simulink model "STM32Inverter2Motor"  (R2025a)
settings: Solver=VariableStepAuto  StartTime=0.0  StopTime=10  RelTol=1e-3
model workspace (MAT data in the model file):
  CT_AmpersPerLSB = 0.0515718
  InverterVdc = 440
  Max_ADC_CNT = 4096
  MotorBaseCurrent = 70
  MotorKe = 43.834
  MotorLd = 0.000222
  MotorLq = 0.000355
  MotorPoles = 4
  MotorRs = 0.126
  PID_ramp = 1000
  PI_params_idKi = 1.5
  PI_params_idKp = 1.92
  PI_params_iqKi = 1.5
  PI_params_iqKp = 2.4
  Ts = 4.34782608696e-05
libraries: simulink x2, slpidlib x2, mcbplantlib x1, autolibpmsminterior x1, mcbcontrollergainlib x1, spsRMSLib x1, simulink_extras x1, mcbhdlcontrolslib x1
settings Model: Creator=taiji  LastModifiedBy=taiji
settings DebuggingCC: ParamSuppressDoubleToSinglePrecisionLossMsg=on
settings RTWCC: GenCodeOnly=on  Toolchain=MinGW64 | gmake (64-bit Windows)

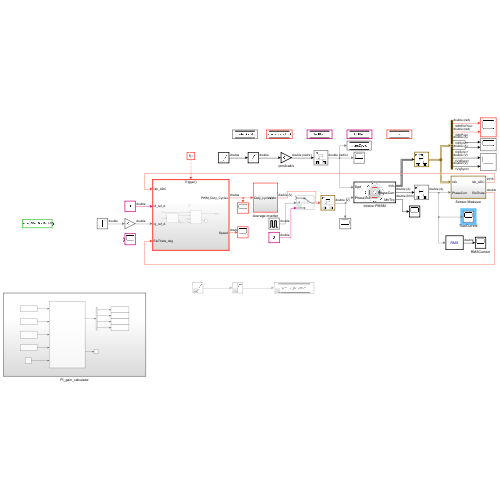
[thumbnail: Simulink's stored preview of the top-level diagram]
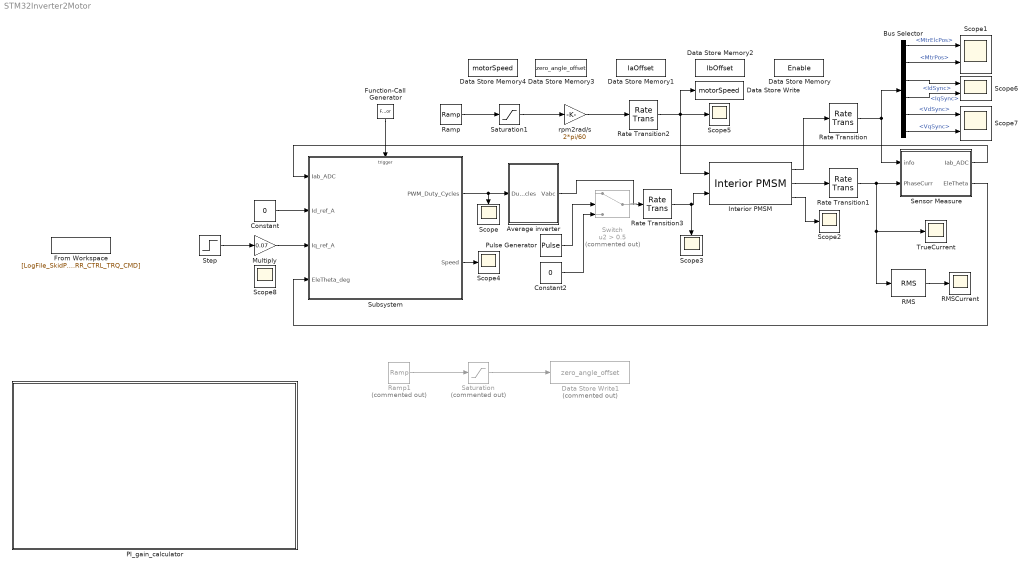
== system STM32Inverter2Motor ==
  Average inverter : Subsystem
  Bus Selector : BusSelector  OutputSignals=MtrElcPos,MtrPos,IdSync,IqSync,VdSync,VqSync
  Constant : Constant  Value=0
  Constant2 : Constant  Value=0
  Data Store Memory : DataStoreMemory  DataStoreName=Enable  WriteAfterWriteMsg=warning  InitialValue=true  ShowAdditionalParam=off  OutDataTypeStr=boolean
  Data Store Memory1 : DataStoreMemory  DataStoreName=IaOffset  WriteAfterWriteMsg=warning  ShowAdditionalParam=off  OutDataTypeStr=boolean
  Data Store Memory2 : DataStoreMemory  DataStoreName=IbOffset  WriteAfterWriteMsg=warning  ShowAdditionalParam=off  OutDataTypeStr=boolean
  Data Store Memory3 : DataStoreMemory  DataStoreName=zero_angle_offset  WriteAfterWriteMsg=warning  InitialValue=36  ShowAdditionalParam=off
  Data Store Memory4 : DataStoreMemory  DataStoreName=motorSpeed  WriteAfterWriteMsg=warning  ShowAdditionalParam=off
  Data Store Write : DataStoreWrite  DataStoreName=motorSpeed  IndexOptions=Index vector (dialog)  Indices=1  OutputSizes=1
  Data Store Write1 : DataStoreWrite  Commented=on  DataStoreName=zero_angle_offset  IndexOptions=Index vector (dialog)  Indices=1  OutputSizes=1
  From Workspace : FromWorkspace  VariableName=[LogFile_SkidPadHiL_TCon_TCoff_0825.Time LogFile_SkidPadHiL_TCon_TCoff_0825.RR_CTRL_TRQ_CMD]  SampleTime=0.001
  Function-Call Generator : FunctionCallGenerator  SampleTime=Ts
  Interior PMSM : autolibpmsminterior/Interior PMSM  port_config=Speed  sim_type=Continuous  Ts=Ts  P=MotorPoles  Rs=MotorRs  Ldq=[MotorLd MotorLq]  KConstText=Back-emf constant (Ke):  lambda_pm=0.0427  Ke=MotorKe  mechanical=[0.33e-3,4.924e-4,0]  idq0=[0 0]  theta_init=0  omega_init=0  KConst=MotorKe  lambda_pm_calc=0.060417  Kt=0.07  RefBlkName='autolibpmsminterior/Interior PMSM'  aMode=5
      settings: LibrarySourceBlock=mcblib/Electrical Systems/Motors/Interior PMSM
  Multiply : Gain  Gain=0.07
  PI_gain_calculator : Subsystem
  Pulse Generator : DiscretePulseGenerator  PulseType=Time based  Period=0.01  PulseWidth=99.99
  RMS : spsRMSLib/RMS  TrueRMS=on  Freq=10  RMSInit=1  Ts=0
  RMSCurrent : Scope
      settings: ActiveDisplayYMinimum=-1  ActiveDisplayYMaximum=1
  Ramp : simulink/Sources/Ramp  slope=100  start=1  InitialOutput=0
  Ramp1 : simulink/Sources/Ramp  Commented=on  slope=36  start=1  InitialOutput=0
  Rate Transition{,1..3} (4 alike) : RateTransition
  Saturation : Saturate  Commented=on  UpperLimit=360  LowerLimit=0
  Saturation1 : Saturate  UpperLimit=600  LowerLimit=0
  Scope{,2..5,8} (6 alike) : Scope
      Scope settings: ActiveDisplayYMinimum=0.15237461254211696  ActiveDisplayYMaximum=0.847625387457883
      Scope2 settings: ActiveDisplayYMinimum=-45.081836654015575  ActiveDisplayYMaximum=14.201489134555768  DataLoggingVariableName=ScopeData2
      Scope3 settings: ActiveDisplayYMinimum=-253.21724341215781  ActiveDisplayYMaximum=253.44594110211258  DataLoggingVariableName=ScopeData3
      Scope4 settings: ActiveDisplayYMinimum=-1  ActiveDisplayYMaximum=1  DataLoggingVariableName=ScopeData2
      Scope5 settings: ActiveDisplayYMinimum=-1  ActiveDisplayYMaximum=1  DataLoggingVariableName=ScopeData9
      Scope8 settings: ActiveDisplayYMinimum=-1  ActiveDisplayYMaximum=1  DataLoggingVariableName=ScopeData14
  Scope1 : Scope  NumInputPorts=2
      settings: ActiveDisplayYMinimum=-1  ActiveDisplayYMaximum=1
  Scope6 : Scope  NumInputPorts=2
  Scope7 : Scope  NumInputPorts=2
      settings: ActiveDisplayYMinimum=-0.8281  ActiveDisplayYMaximum=6.44112  DataLoggingVariableName=ScopeData2
  Sensor Measure : Subsystem
  Step : Step  Time=0.2  After=1000  SampleTime=0
  Subsystem : Subsystem
  Switch : Switch  Commented=on  Criteria=u2 > Threshold  Threshold=0.5  SaturateOnIntegerOverflow=off  InputSameDT=off
  TrueCurrent : Scope
      settings: ActiveDisplayYMinimum=-87.035051528006122  ActiveDisplayYMaximum=87.028426331999526  DataLoggingVariableName=ScopeData7
  rpm2rad/s : Gain  Gain=2*pi/60
  wires:
  Interior PMSM/1 -> Rate Transition/1
  Interior PMSM/2 -> Rate Transition1/1
  Average inverter/1(Vabc) -> Rate Transition3/1
  Rate Transition/1 -> Sensor Measure/1(info), Bus Selector/1
  Rate Transition1/1 -> RMS/1, TrueCurrent/1, Sensor Measure/2(PhaseCurr)
  Bus Selector/1 -> Scope1/1  "<MtrElcPos>"
  Rate Transition3/1 -> Interior PMSM/2, Scope3/1
  Function-Call Generator/1 -> Subsystem/Trigger
  Subsystem/1(PWM_Duty_Cycles) -> Average inverter/1(Duty_cycles), Scope/1
  Interior PMSM/3 -> Scope2/1
  RMS/1 -> RMSCurrent/1
  Subsystem/2(Speed) -> Scope4/1
  Ramp/1 -> Saturation1/1
  Rate Transition2/1 -> Interior PMSM/1, Data Store Write/1, Scope5/1
  rpm2rad/s/1 -> Rate Transition2/1
  Bus Selector/2 -> Scope1/2  "<MtrPos>"
  Bus Selector/3 -> Scope6/1  "<IdSync>"
  Bus Selector/4 -> Scope6/2  "<IqSync>"
  Bus Selector/5 -> Scope7/1  "<VdSync>"
  Bus Selector/6 -> Scope7/2  "<VqSync>"
  Constant/1 -> Subsystem/2(Id_ref_A)
  Multiply/1 -> Subsystem/3(Iq_ref_A)
  Ramp1/1 -> Saturation/1
  Sensor Measure/2(EleTheta) -> Subsystem/4(EleTheta_deg)
  Sensor Measure/1(Iab_ADC) -> Subsystem/1(Iab_ADC)
  Saturation/1 -> Data Store Write1/1
  Saturation1/1 -> rpm2rad/s/1
  Switch/1 -> ?
  Pulse Generator/1 -> Switch/2
  Constant2/1 -> Switch/3
  Step/1 -> Multiply/1

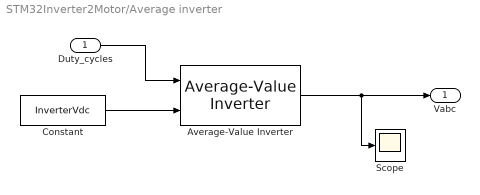
== system STM32Inverter2Motor/Average inverter ==
  Duty_cycles : Inport
  Average-Value Inverter : mcbplantlib/Average-Value Inverter
      settings: LibrarySourceBlock=mcblib/Electrical Systems/Inverters/Average-Value Inverter
  Constant : Constant  Value=InverterVdc
  Scope : Scope
      settings: ActiveDisplayYMinimum=-313.23796592607141  ActiveDisplayYMaximum=350.5718291969751  DataLoggingVariableName=ScopeData6
  Vabc : Outport
  wires:
  Duty_cycles/1 -> Average-Value Inverter/1
  Constant/1 -> Average-Value Inverter/2
  Average-Value Inverter/1 -> Scope/1, Vabc/1

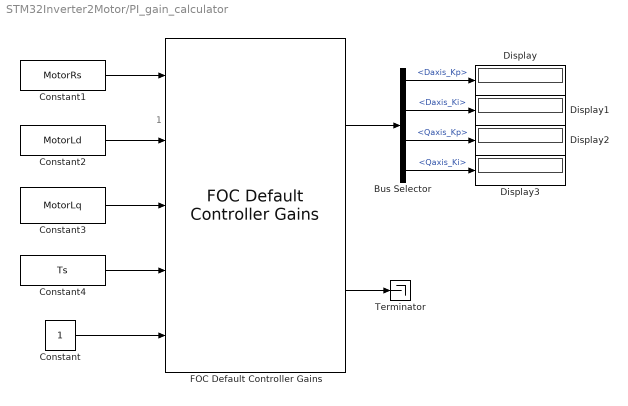
== system STM32Inverter2Motor/PI_gain_calculator ==
  note: 1
  Bus Selector : BusSelector  OutputSignals=Daxis_Kp,Daxis_Ki,Qaxis_Kp,Qaxis_Ki
  Constant : Constant
  Constant1 : Constant  Value=MotorRs
  Constant2 : Constant  Value=MotorLd
  Constant3 : Constant  Value=MotorLq
  Constant4 : Constant  Value=Ts  VectorParams1D=off
  Display{,1..3} (4 alike) : Display
  FOC Default Controller Gains : mcbcontrollergainlib/FOC Default Controller Gains  ControllerGainType=Empirical method  motorSelection=PMSM  unitType=SI Unit  outCurrentControlGain=on  outFWCGain=off  outSpeedControlGain=off  externalDelay=off  currentSensorDelay=50e-6  speedSensorDelay=50e-6  speedFilterDelay=0.02
      settings: LibrarySourceBlock=mcblib/Controls/Controllers/FOC Default Controller Gains
  Terminator : Terminator
  wires:
  FOC Default Controller Gains/1 -> Bus Selector/1
  FOC Default Controller Gains/2 -> Terminator/1
  Constant4/1 -> FOC Default Controller Gains/4
  Constant3/1 -> FOC Default Controller Gains/3
  Constant2/1 -> FOC Default Controller Gains/2
  Constant1/1 -> FOC Default Controller Gains/1
  Constant/1 -> FOC Default Controller Gains/5
  Bus Selector/1 -> Display/1  "<Daxis_Kp>"
  Bus Selector/2 -> Display1/1  "<Daxis_Ki>"
  Bus Selector/3 -> Display2/1  "<Qaxis_Kp>"
  Bus Selector/4 -> Display3/1  "<Qaxis_Ki>"

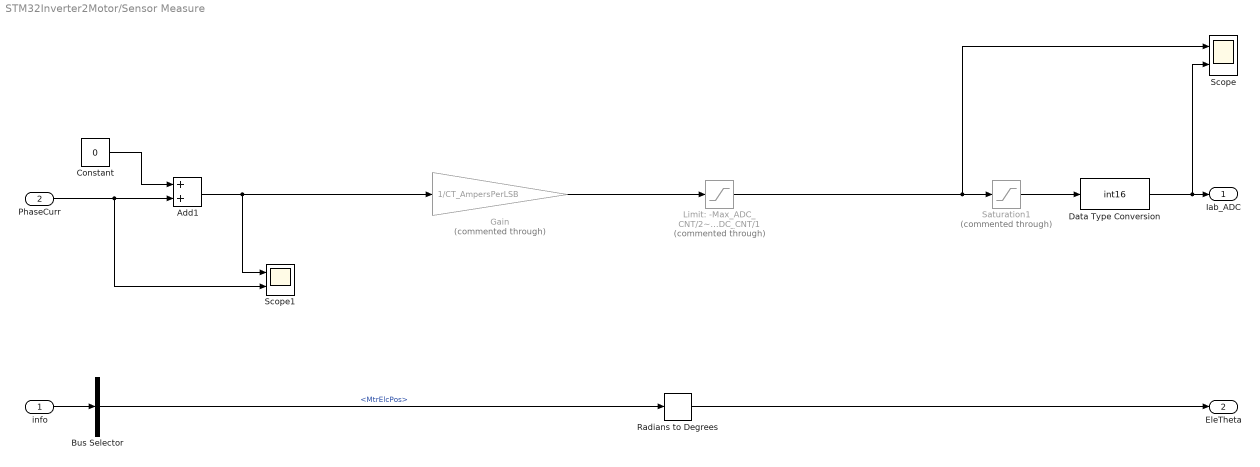
== system STM32Inverter2Motor/Sensor Measure ==
  info : Inport
  PhaseCurr : Inport  Port=2
  Add1 : Sum
  Bus Selector : BusSelector  OutputSignals=MtrElcPos
  Constant : Constant  Value=0
  Data Type Conversion : DataTypeConversion  OutDataTypeStr=int16  SaturateOnIntegerOverflow=off  RndMeth=Floor
  Gain : Gain  Commented=through  Gain=1/CT_AmpersPerLSB
  Limit: -Max_ADC_CNT/2~Max_ADC_CNT/1 : Saturate  Commented=through  UpperLimit=Max_ADC_CNT/2  LowerLimit=-Max_ADC_CNT/2
  Radians to Degrees : simulink_extras/Transformations/Radians to Degrees
  Saturation1 : Saturate  Commented=through  UpperLimit=Max_ADC_CNT  LowerLimit=0
  Scope : Scope  NumInputPorts=2
      settings: ActiveDisplayYMinimum=-2386.1587583821911  ActiveDisplayYMaximum=2388.3518252217932
  Scope1 : Scope  NumInputPorts=2
      settings: ActiveDisplayYMinimum=-2421.1249474633973  ActiveDisplayYMaximum=2418.5627534419714
  Iab_ADC : Outport
  EleTheta : Outport  Port=2
  wires:
  Gain/1 -> Limit: -Max_ADC_CNT/2~Max_ADC_CNT/1/1
  Saturation1/1 -> Data Type Conversion/1
  Limit: -Max_ADC_CNT/2~Max_ADC_CNT/1/1 -> Scope/1, Saturation1/1
  Add1/1 -> Scope1/1, Gain/1
  Data Type Conversion/1 -> Scope/2, Iab_ADC/1
  info/1 -> Bus Selector/1
  Bus Selector/1 -> Radians to Degrees/1  "<MtrElcPos>"
  PhaseCurr/1 -> Scope1/2, Add1/2
  Constant/1 -> Add1/1
  Radians to Degrees/1 -> EleTheta/1

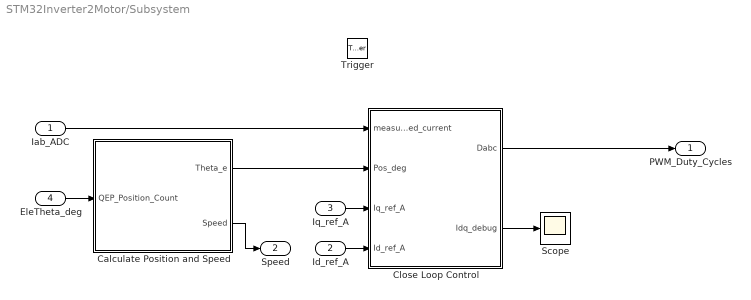
== system STM32Inverter2Motor/Subsystem ==
  Iab_ADC : Inport
  Id_ref_A : Inport  Port=2
  Iq_ref_A : Inport  Port=3
  EleTheta_deg : Inport  Port=4
  Trigger : TriggerPort  TriggerType=function-call  VariantControl=(inherit)  PortDimensions=1
  Calculate Position and Speed : Subsystem
  Close Loop Control : Subsystem
  Scope : Scope
      settings: ActiveDisplayYMinimum=-1  ActiveDisplayYMaximum=1  DataLoggingVariableName=ScopeData8
  PWM_Duty_Cycles : Outport
  Speed : Outport  Port=2
  wires:
  Calculate Position and Speed/1(Theta_e) -> Close Loop Control/2(Pos_deg)
  Iab_ADC/1 -> Close Loop Control/1(measured_current)
  Close Loop Control/1(Dabc) -> PWM_Duty_Cycles/1
  Close Loop Control/2(Idq_debug) -> Scope/1
  Calculate Position and Speed/2(Speed) -> Speed/1
  EleTheta_deg/1 -> Calculate Position and Speed/1(QEP_Position_Count)
  Iq_ref_A/1 -> Close Loop Control/3(Iq_ref_A)
  Id_ref_A/1 -> Close Loop Control/4(Id_ref_A)

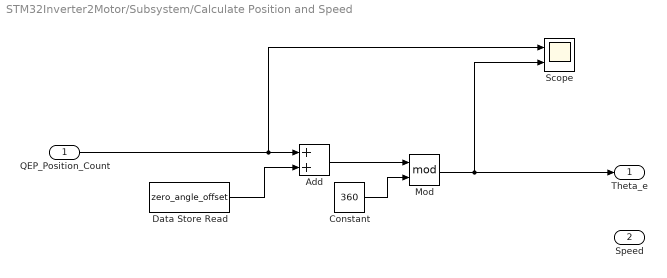
== system STM32Inverter2Motor/Subsystem/Calculate Position and Speed ==
  QEP_Position_Count : Inport
  Add : Sum
  Constant : Constant  Value=360
  Data Store Read : DataStoreRead  DataStoreName=zero_angle_offset  IndexOptions=Index vector (dialog)  Indices=1  OutputSizes=1
  Mod : Math  Operator=mod
  Scope : Scope  NumInputPorts=2
      settings: ActiveDisplayYMinimum=-1  ActiveDisplayYMaximum=1
  Theta_e : Outport
  Speed : Outport  Port=2
  wires:
  QEP_Position_Count/1 -> Scope/1, Add/1
  Constant/1 -> Mod/2
  Add/1 -> Mod/1
  Data Store Read/1 -> Add/2
  Mod/1 -> Theta_e/1, Scope/2

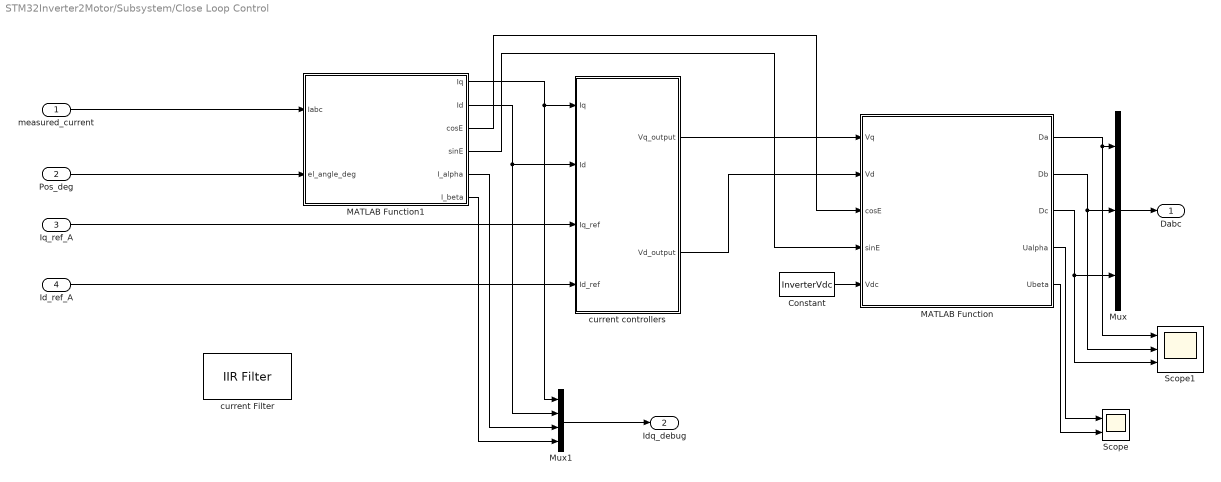
== system STM32Inverter2Motor/Subsystem/Close Loop Control ==
  measured_current : Inport
  Pos_deg : Inport  Port=2
  Iq_ref_A : Inport  Port=3
  Id_ref_A : Inport  Port=4
  Constant : Constant  Value=InverterVdc
  MATLAB Function : MATLAB Function  TreatAsAtomicUnit=on
  MATLAB Function1 : MATLAB Function  TreatAsAtomicUnit=on
  Mux : Mux  Inputs=3
  Mux1 : Mux
  Scope : Scope  NumInputPorts=2
      settings: ActiveDisplayYMinimum=-1  ActiveDisplayYMaximum=1  DataLoggingVariableName=ScopeData11
  Scope1 : Scope  NumInputPorts=3
      settings: ActiveDisplayYMinimum=-0.12499999999999997  ActiveDisplayYMaximum=1.125
  current Filter : mcbhdlcontrolslib/IIR Filter  VariantControl=Low Pass Filter  VariantSelect=Low-pass  FilterConstantInputType=Specify via dialog  Filter_constant=0.532  advancedSettings=on  Ts=Ts  cutOff_freq=4161.1536
      settings: LibrarySourceBlock=mcbhdllib/Signal Management/IIR Filter
  current controllers : Subsystem
  Dabc : Outport
  Idq_debug : Outport  Port=2
  wires:
  MATLAB Function1/2(Id) -> Mux1/2, current controllers/2(Id)
  Iq_ref_A/1 -> current controllers/3(Iq_ref)
  Mux/1 -> Dabc/1
  MATLAB Function1/1(Iq) -> Mux1/1, current controllers/1(Iq)
  Id_ref_A/1 -> current controllers/4(Id_ref)
  Mux1/1 -> Idq_debug/1
  MATLAB Function/1(Da) -> Mux/1, Scope1/1
  MATLAB Function/2(Db) -> Mux/2, Scope1/2
  MATLAB Function/3(Dc) -> Mux/3, Scope1/3
  measured_current/1 -> MATLAB Function1/1(Iabc)
  Pos_deg/1 -> MATLAB Function1/2(el_angle_deg)
  Constant/1 -> MATLAB Function/5(Vdc)
  current controllers/1(Vq_output) -> MATLAB Function/1(Vq)
  current controllers/2(Vd_output) -> MATLAB Function/2(Vd)
  MATLAB Function1/3(cosE) -> MATLAB Function/3(cosE)
  MATLAB Function1/4(sinE) -> MATLAB Function/4(sinE)
  MATLAB Function1/5(I_alpha) -> Mux1/3
  MATLAB Function1/6(I_beta) -> Mux1/4
  MATLAB Function/4(Ualpha) -> Scope/1
  MATLAB Function/5(Ubeta) -> Scope/2

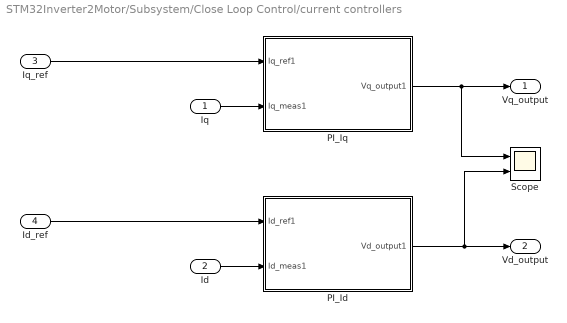
== system STM32Inverter2Motor/Subsystem/Close Loop Control/current controllers ==
  Iq : Inport
  Id : Inport  Port=2
  Iq_ref : Inport  Port=3
  Id_ref : Inport  Port=4
  PI_Id : Subsystem
  PI_Iq : Subsystem
  Scope : Scope  NumInputPorts=2
      settings: ActiveDisplayYMinimum=-1  ActiveDisplayYMaximum=1  DataLoggingVariableName=ScopeData12
  Vq_output : Outport
  Vd_output : Outport  Port=2
  wires:
  PI_Iq/1(Vq_output1) -> Vq_output/1, Scope/1
  PI_Id/1(Vd_output1) -> Scope/2, Vd_output/1
  Id/1 -> PI_Id/2(Id_meas1)
  Iq/1 -> PI_Iq/2(Iq_meas1)
  Iq_ref/1 -> PI_Iq/1(Iq_ref1)
  Id_ref/1 -> PI_Id/1(Id_ref1)

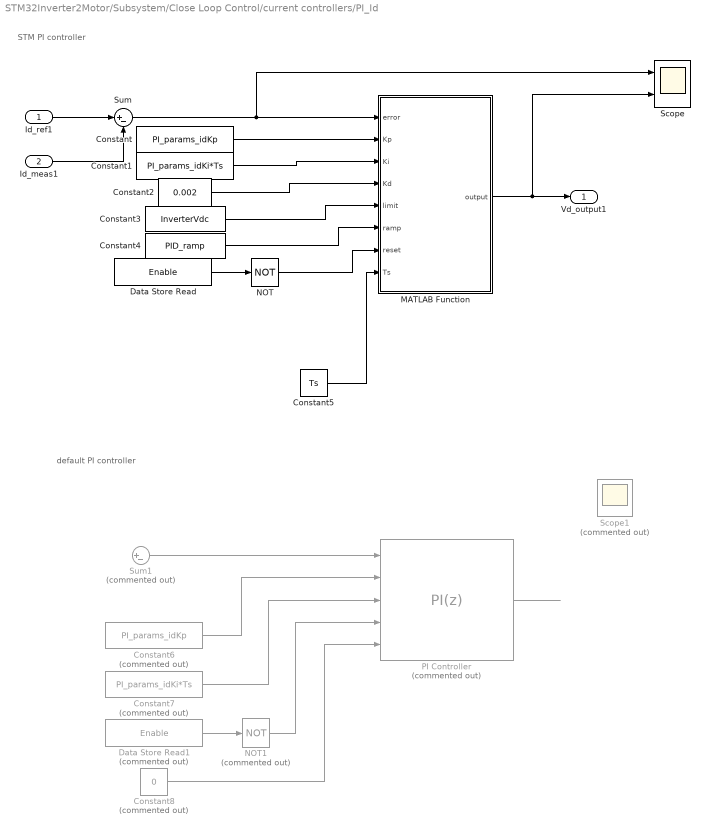
== system STM32Inverter2Motor/Subsystem/Close Loop Control/current controllers/PI_Id ==
  note: STM PI controller
  note: default PI controller
  Id_ref1 : Inport
  Id_meas1 : Inport  Port=2
  Constant : Constant  Value=PI_params_idKp
  Constant1 : Constant  Value=PI_params_idKi*Ts
  Constant2 : Constant  Value=0.002
  Constant3 : Constant  Value=InverterVdc
  Constant4 : Constant  Value=PID_ramp
  Constant5 : Constant  Value=Ts
  Constant6 : Constant  Commented=on  Value=PI_params_idKp
  Constant7 : Constant  Commented=on  Value=PI_params_idKi*Ts
  Constant8 : Constant  Commented=on  Value=0
  Data Store Read : DataStoreRead  DataStoreName=Enable  IndexOptions=Index vector (dialog)  Indices=1  OutputSizes=1
  Data Store Read1 : DataStoreRead  Commented=on  DataStoreName=Enable  IndexOptions=Index vector (dialog)  Indices=1  OutputSizes=1
  MATLAB Function : MATLAB Function  TreatAsAtomicUnit=on
  NOT : Logic  Operator=NOT  IconShape=distinctive  AllPortsSameDT=off  OutDataTypeStr=boolean
  NOT1 : Logic  Commented=on  Operator=NOT  IconShape=distinctive  AllPortsSameDT=off  OutDataTypeStr=boolean
  PI Controller : slpidlib/PID Controller  Commented=on  Controller=PI  Form=Parallel  TimeDomain=Discrete-time  UseExternalTs=off  SampleTime=-1  IntegratorMethod=Forward Euler  FilterMethod=Forward Euler  ControllerParametersSource=external  P=1  I=1  UseKiTs=on  D=0  UseExternalDerivativeSource=off  N=100  UseFilter=on  TunerSelectOption=Transfer Function Based (PID Tuner App)  InitialConditionSource=external  InitialConditionForIntegrator=0  InitialConditionForFilter=0  DifferentiatorICPrevScaledInput=0  ExternalReset=level  TrackingMode=off  Kt=1  LimitOutput=on  SatLimitsSource=internal  UpperSaturationLimit=InverterVdc  LowerSaturationLimit=-InverterVdc  LinearizeAsGain=on  AntiWindupMode=clamping  Kb=1  LimitIntegrator=on  UpperIntegratorSaturationLimit=InverterVdc  LowerIntegratorSaturationLimit=-InverterVdc  RndMeth=Simplest  POutMin=[]  POutMax=[]  IOutMin=[]  IOutMax=[]  DOutMin=[]  DOutMax=[]  NOutMin=[]  NOutMax=[]  SumOutMin=[]  SumOutMax=[]  SaturationOutDataTypeStr=Inherit: Inherit via back propagation  SaturationOutMin=[]  SaturationOutMax=[]  PParamMin=[]  PParamMax=[]  IParamMin=[]  IParamMax=[]  DParamMin=[]  DParamMax=[]  NParamMin=[]  NParamMax=[]  KbParamMin=[]  KbParamMax=[]  KtParamMin=[]  KtParamMax=[]  KbOutMin=[]  KbOutMax=[]  KtOutMin=[]  KtOutMax=[]  IntegratorOutMin=[]  IntegratorOutMax=[]  FilterOutMin=[]  FilterOutMax=[]  SumI1OutMin=[]  SumI1OutMax=[]  SumI2OutMin=[]  SumI2OutMax=[]  SumI3OutMin=[]  SumI3OutMax=[]  SumI4OutMin=[]  SumI4OutMax=[]  SumDOutMin=[]  SumDOutMax=[]  DifferentiatorOutMin=[]  DifferentiatorOutMax=[]  FilterDiffOutCoefMin=[]  FilterDiffOutCoefMax=[]  ReciprocalOutMin=[]  ReciprocalOutMax=[]  SumDenOutMin=[]  SumDenOutMax=[]  SumNumOutMin=[]  SumNumOutMax=[]  DivideOutMin=[]  DivideOutMax=[]  UdiffTsProdOutMin=[]  UdiffTsProdOutMax=[]  NTsProdOutMin=[]  NTsProdOutMax=[]  UintegralTsProdOutMin=[]  UintegralTsProdOutMax=[]  UngainTsProdOutMin=[]  UngainTsProdOutMax=[]  ClampingZeroOutDataTypeStr=Inherit: Inherit via back propagation  ClampingZeroOutMin=[]  ClampingZeroOutMax=[]  FilterDenConstantOutDataTypeStr=Inherit: Inherit via back propagation  FilterDenConstantOutMin=[]  FilterDenConstantOutMax=[]  PCopyOutDataTypeStr=Inherit: Inherit via back propagation  PCopyOutMin=[]  PCopyOutMax=[]  NCopyOutDataTypeStr=Inherit: Inherit via back propagation  NCopyOutMin=[]  NCopyOutMax=[]  IntegratorContinuousStateAttributes=''  IntegratorStateMustResolveToSignalObject=off  IntegratorRTWStateStorageClass=Auto  FilterContinuousStateAttributes=''  FilterStateMustResolveToSignalObject=off  FilterRTWStateStorageClass=Auto  ParallelPVariant=ExternalParameters  IdealPVariant=Disabled  IVariant=ExternalParameters  DVariant=Disabled  IntegratorVariant=Discrete  SatVariant=Enabled  AWVariant=DiscClampingParallel  PCopyVariant=Disabled  TRVariant=Disabled  FdbkBlocksVariant=Forward  IdealPFdbkVariant=Disabled  SatFdbkVariant=Disabled  DerivativeFilterVariant=Disabled  NVariant=Disabled  NCopyVariant=Disabled_SignalSpec  FilterICVariant=Disabled  IntegratorICVariant=ExternalICs  ExternalResetVariant=ExternalReset  TRSumVariant=Passthrough  SumFdbkVariant=Disabled  SumVariant=Sum_PI  TsampFilterVariant=InternalTs  TsampNgainVariant=Passthrough  TsampIntegralVariant=Disabled_SignalSpec  ExternalSaturationOutDataTypeStr=Inherit: Same as second input  DerivativeSourceVariant=Disabled  PreIntVariant=InternalPreInt
  Scope : Scope  NumInputPorts=2
      settings: ActiveDisplayYMinimum=-4.2718355978255875  ActiveDisplayYMaximum=8.44652038043029  DataLoggingVariableName=ScopeData10
  Scope1 : Scope  Commented=on  NumInputPorts=3
      settings: ActiveDisplayYMinimum=-1  ActiveDisplayYMaximum=1  DataLoggingVariableName=ScopeData15
  Sum : Sum  Inputs=|+-
  Sum1 : Sum  Commented=on  Inputs=|+-
  Vd_output1 : Outport
  wires:
  Id_ref1/1 -> Sum/1
  Constant2/1 -> MATLAB Function/4(Kd)
  NOT/1 -> MATLAB Function/7(reset)
  Id_meas1/1 -> Sum/2
  Constant1/1 -> MATLAB Function/3(Ki)
  Constant/1 -> MATLAB Function/2(Kp)
  Data Store Read/1 -> NOT/1
  Sum/1 -> Scope/1, MATLAB Function/1(error)
  Constant3/1 -> MATLAB Function/5(limit)
  Constant4/1 -> MATLAB Function/6(ramp)
  Constant5/1 -> MATLAB Function/8(Ts)
  MATLAB Function/1(output) -> Vd_output1/1, Scope/2
  ? -> Scope1/2, Sum1/2
  Data Store Read1/1 -> NOT1/1
  Constant7/1 -> PI Controller/3
  ? -> Scope1/1, Sum1/1
  Constant6/1 -> PI Controller/2
  Constant8/1 -> PI Controller/5
  NOT1/1 -> PI Controller/4
  Sum1/1 -> PI Controller/1
  PI Controller/1 -> ?

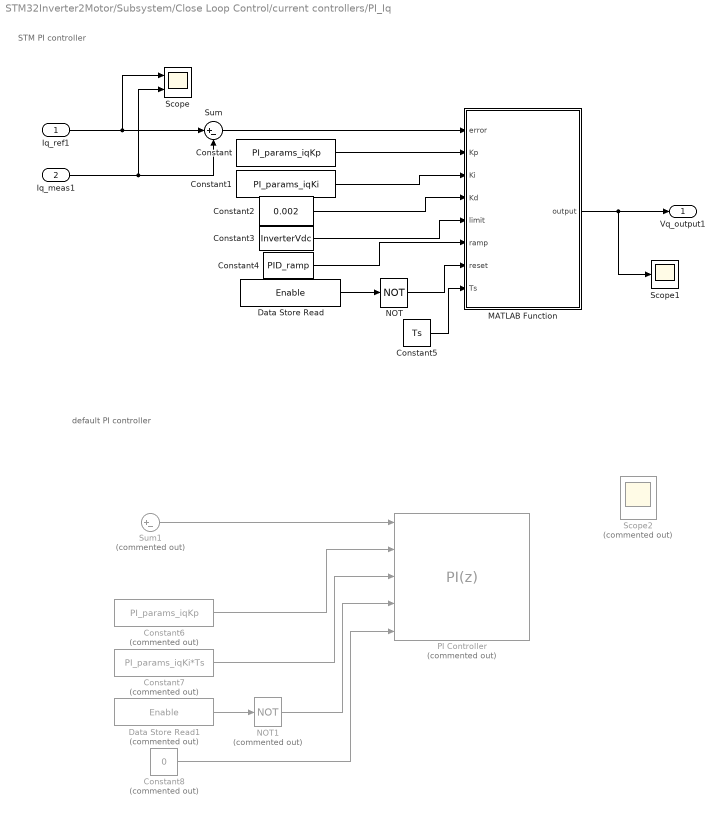
== system STM32Inverter2Motor/Subsystem/Close Loop Control/current controllers/PI_Iq ==
  note: STM PI controller
  note: default PI controller
  Iq_ref1 : Inport
  Iq_meas1 : Inport  Port=2
  Constant : Constant  Value=PI_params_iqKp
  Constant1 : Constant  Value=PI_params_iqKi
  Constant2 : Constant  Value=0.002
  Constant3 : Constant  Value=InverterVdc
  Constant4 : Constant  Value=PID_ramp
  Constant5 : Constant  Value=Ts
  Constant6 : Constant  Commented=on  Value=PI_params_iqKp
  Constant7 : Constant  Commented=on  Value=PI_params_iqKi*Ts
  Constant8 : Constant  Commented=on  Value=0
  Data Store Read : DataStoreRead  DataStoreName=Enable  IndexOptions=Index vector (dialog)  Indices=1  OutputSizes=1
  Data Store Read1 : DataStoreRead  Commented=on  DataStoreName=Enable  IndexOptions=Index vector (dialog)  Indices=1  OutputSizes=1
  MATLAB Function : MATLAB Function  TreatAsAtomicUnit=on
  NOT : Logic  Operator=NOT  IconShape=distinctive  AllPortsSameDT=off  OutDataTypeStr=boolean
  NOT1 : Logic  Commented=on  Operator=NOT  IconShape=distinctive  AllPortsSameDT=off  OutDataTypeStr=boolean
  PI Controller : slpidlib/PID Controller  Commented=on  Controller=PI  Form=Parallel  TimeDomain=Discrete-time  UseExternalTs=off  SampleTime=-1  IntegratorMethod=Forward Euler  FilterMethod=Forward Euler  ControllerParametersSource=external  P=1  I=1  UseKiTs=on  D=0  UseExternalDerivativeSource=off  N=100  UseFilter=on  TunerSelectOption=Transfer Function Based (PID Tuner App)  InitialConditionSource=external  InitialConditionForIntegrator=0  InitialConditionForFilter=0  DifferentiatorICPrevScaledInput=0  ExternalReset=level  TrackingMode=off  Kt=1  LimitOutput=on  SatLimitsSource=internal  UpperSaturationLimit=InverterVdc  LowerSaturationLimit=-InverterVdc  LinearizeAsGain=on  AntiWindupMode=clamping  Kb=1  LimitIntegrator=on  UpperIntegratorSaturationLimit=InverterVdc  LowerIntegratorSaturationLimit=-InverterVdc  RndMeth=Simplest  POutMin=[]  POutMax=[]  IOutMin=[]  IOutMax=[]  DOutMin=[]  DOutMax=[]  NOutMin=[]  NOutMax=[]  SumOutMin=[]  SumOutMax=[]  SaturationOutDataTypeStr=Inherit: Inherit via back propagation  SaturationOutMin=[]  SaturationOutMax=[]  PParamMin=[]  PParamMax=[]  IParamMin=[]  IParamMax=[]  DParamMin=[]  DParamMax=[]  NParamMin=[]  NParamMax=[]  KbParamMin=[]  KbParamMax=[]  KtParamMin=[]  KtParamMax=[]  KbOutMin=[]  KbOutMax=[]  KtOutMin=[]  KtOutMax=[]  IntegratorOutMin=[]  IntegratorOutMax=[]  FilterOutMin=[]  FilterOutMax=[]  SumI1OutMin=[]  SumI1OutMax=[]  SumI2OutMin=[]  SumI2OutMax=[]  SumI3OutMin=[]  SumI3OutMax=[]  SumI4OutMin=[]  SumI4OutMax=[]  SumDOutMin=[]  SumDOutMax=[]  DifferentiatorOutMin=[]  DifferentiatorOutMax=[]  FilterDiffOutCoefMin=[]  FilterDiffOutCoefMax=[]  ReciprocalOutMin=[]  ReciprocalOutMax=[]  SumDenOutMin=[]  SumDenOutMax=[]  SumNumOutMin=[]  SumNumOutMax=[]  DivideOutMin=[]  DivideOutMax=[]  UdiffTsProdOutMin=[]  UdiffTsProdOutMax=[]  NTsProdOutMin=[]  NTsProdOutMax=[]  UintegralTsProdOutMin=[]  UintegralTsProdOutMax=[]  UngainTsProdOutMin=[]  UngainTsProdOutMax=[]  ClampingZeroOutDataTypeStr=Inherit: Inherit via back propagation  ClampingZeroOutMin=[]  ClampingZeroOutMax=[]  FilterDenConstantOutDataTypeStr=Inherit: Inherit via back propagation  FilterDenConstantOutMin=[]  FilterDenConstantOutMax=[]  PCopyOutDataTypeStr=Inherit: Inherit via back propagation  PCopyOutMin=[]  PCopyOutMax=[]  NCopyOutDataTypeStr=Inherit: Inherit via back propagation  NCopyOutMin=[]  NCopyOutMax=[]  IntegratorContinuousStateAttributes=''  IntegratorStateMustResolveToSignalObject=off  IntegratorRTWStateStorageClass=Auto  FilterContinuousStateAttributes=''  FilterStateMustResolveToSignalObject=off  FilterRTWStateStorageClass=Auto  ParallelPVariant=ExternalParameters  IdealPVariant=Disabled  IVariant=ExternalParameters  DVariant=Disabled  IntegratorVariant=Discrete  SatVariant=Enabled  AWVariant=DiscClampingParallel  PCopyVariant=Disabled  TRVariant=Disabled  FdbkBlocksVariant=Forward  IdealPFdbkVariant=Disabled  SatFdbkVariant=Disabled  DerivativeFilterVariant=Disabled  NVariant=Disabled  NCopyVariant=Disabled_SignalSpec  FilterICVariant=Disabled  IntegratorICVariant=ExternalICs  ExternalResetVariant=ExternalReset  TRSumVariant=Passthrough  SumFdbkVariant=Disabled  SumVariant=Sum_PI  TsampFilterVariant=InternalTs  TsampNgainVariant=Passthrough  TsampIntegralVariant=Disabled_SignalSpec  ExternalSaturationOutDataTypeStr=Inherit: Same as second input  DerivativeSourceVariant=Disabled  PreIntVariant=InternalPreInt
      settings: LibrarySourceBlock=mcblib/Controls/Controllers/PI Controller
  Scope : Scope  NumInputPorts=2
      settings: ActiveDisplayYMinimum=-8.9999999999999982  ActiveDisplayYMaximum=81  DataLoggingVariableName=ScopeData4
  Scope1 : Scope
      settings: ActiveDisplayYMinimum=-1  ActiveDisplayYMaximum=1  DataLoggingVariableName=ScopeData5
  Scope2 : Scope  Commented=on  NumInputPorts=2
      settings: ActiveDisplayYMinimum=-1.819404069767443  ActiveDisplayYMaximum=10.583720930232559  DataLoggingVariableName=ScopeData13
  Sum : Sum  Inputs=|+-
  Sum1 : Sum  Commented=on  Inputs=|+-
  Vq_output1 : Outport
  wires:
  Iq_ref1/1 -> Scope/1, Sum/1
  Constant2/1 -> MATLAB Function/4(Kd)
  NOT/1 -> MATLAB Function/7(reset)
  Iq_meas1/1 -> Scope/2, Sum/2
  Constant1/1 -> MATLAB Function/3(Ki)
  Constant/1 -> MATLAB Function/2(Kp)
  MATLAB Function/1(output) -> Vq_output1/1, Scope1/1
  Data Store Read/1 -> NOT/1
  Sum/1 -> MATLAB Function/1(error)
  Constant3/1 -> MATLAB Function/5(limit)
  Constant4/1 -> MATLAB Function/6(ramp)
  Constant5/1 -> MATLAB Function/8(Ts)
  Data Store Read1/1 -> NOT1/1
  Constant7/1 -> PI Controller/3
  NOT1/1 -> PI Controller/4
  Constant8/1 -> PI Controller/5
  Constant6/1 -> PI Controller/2
  Sum1/1 -> PI Controller/1

== matlab function STM32Inverter2Motor/Subsystem/Close Loop Control/MATLAB Function1 ==
  data: Iq output; Iabc input; Id output; el_angle_deg input; cosE output; sinE output; I_alpha output; I_beta output
function [Iq, Id, cosE, sinE, I_alpha, I_beta] = idq_cal(Iabc, el_angle_deg)

cosE = cosd(el_angle_deg);
sinE = sind(el_angle_deg);

mid_current = (Iabc(1) + Iabc(2) + Iabc(3)) / 3.0;

a = Iabc(1) - mid_current;
b = Iabc(2) - mid_current;
I_alpha=a;
I_beta=0.57735026919*(2*b+a);

Iq = -sind(el_angle_deg)*I_alpha+cosd(el_angle_deg)*I_beta;
Id = cosd(el_angle_deg)*I_alpha+sind(el_angle_deg)*I_beta;

== matlab function STM32Inverter2Motor/Subsystem/Close Loop Control/current controllers/PI_Iq/MATLAB Function ==
  data: error input; output output; Kp input; Ki input; Kd input; limit input; ramp input; reset input; Ts input
function output = pid_controller(error, Kp, Ki, Kd, limit, ramp, reset, Ts)
proportional = Kp * error;
persistent error_prev;
persistent output_prev;
persistent integral_prev;

if isempty(error_prev)
    error_prev = 0;
    output_prev = 0;
	integral_prev = 0;
end

if reset == true
    error_prev = 0;
	output_prev = 0;
	integral_prev = 0;
end

% Tustin 散点积分（I环）
integral = integral_prev + Ki*Ts*0.5*(error + error_prev);
integral = sat(integral, -limit, limit);
% D环（微分环节）
derivative = Kd*(error - error_prev)/Ts;

% 将P,I,D三环的计算值加起来
output = proportional + integral + derivative;
output = sat(output, -limit, limit);

if(ramp > 0)
    % 对PID的变化速率进行限制
    output_rate = (output - output_prev)/Ts;
    if (output_rate > ramp)
        output = output_prev + ramp*Ts;
    elseif (output_rate < -ramp)
        output = output_prev - ramp*Ts;
    end
end
% 保存值（为了下一次循环）
if not (output == limit || output == -limit)        
    integral_prev = integral;
end
output_prev = output;
error_prev = error;

== matlab function STM32Inverter2Motor/Subsystem/Close Loop Control/current controllers/PI_Id/MATLAB Function ==
  data: error input; output output; Kp input; Ki input; Kd input; limit input; ramp input; reset input; Ts input
function output = pid_controller(error, Kp, Ki, Kd, limit, ramp, reset, Ts)
proportional = Kp * error;
persistent error_prev;
persistent output_prev;
persistent integral_prev;

if isempty(error_prev)
    error_prev = 0;
    output_prev = 0;
	integral_prev = 0;
end

if reset == true
    error_prev = 0;
	output_prev = 0;
	integral_prev = 0;
end

% Tustin 散点积分（I环）
integral = integral_prev + Ki*0.5*(error + error_prev);
integral = sat(integral, -limit, limit);
% D环（微分环节）
derivative = Kd*(error - error_prev)/Ts;

% 将P,I,D三环的计算值加起来
output = proportional + integral + derivative;
output = sat(output, -limit, limit);

if(ramp > 0)
    % 对PID的变化速率进行限制
    output_rate = (output - output_prev)/Ts;
    if (output_rate > ramp)
        output = output_prev + ramp*Ts;
    elseif (output_rate < -ramp)
        output = output_prev - ramp*Ts;
    end
end
% 保存值（为了下一次循环）
if not (output == limit || output == -limit)        
    integral_prev = integral;
end
output_prev = output;
error_prev = error;

== matlab function STM32Inverter2Motor/Subsystem/Close Loop Control/MATLAB Function ==
  data: Vq input; Vd input; Da output; Db output; Dc output; cosE input; sinE input; Vdc input; Ualpha output; Ubeta output
function [Da, Db, Dc, Ualpha, Ubeta]= middle_clamp_modu(Vq, Vd, cosE, sinE, Vdc)
    Ualpha =  cosE * Vd + -sinE * Vq; % d-axis align with alpha-axis
    Ubeta =  sinE * Vd + cosE * Vq;
    % Ualpha =  sinE * Vd + cosE * Vq; % q-axis align with alpha-axis
    % Ubeta =  -cosE * Vd + sinE * Vq;
    Ua = Ualpha;
    Ub = -0.5 * Ualpha + 0.86602540378 * Ubeta;
    Uc = -0.5 * Ualpha - 0.86602540378 * Ubeta;
    Ua = sat((Ua/Vdc+1)/2, 0, 1);
    Ub = sat((Ub/Vdc+1)/2, 0, 1);
    Uc = sat((Uc/Vdc+1)/2, 0, 1);
    center = 0.5;
    % // discussed here: https://community.simplefoc.com/t/embedded-world-2023-stm32-cordic-co-processor/3107/165?u=cosEndas1
    % // a bit more info here: https://microchipdeveloper.com/mct5001:which-zsm-is-best
    % // Midpoint Clamp
    Umin = min(Ua, min(Ub, Uc));
    Umax = max(Ua, max(Ub, Uc));
    center = center - (Umax+Umin) / 2;
    Da = Ua + center;
    Db = Ub + center;
    Dc = Uc + center; 
end
